simulink model "yunkongkaihuan"  (R2018a)
settings: Solver=VariableStepAuto  StartTime=0.0  StopTime=1  MaxStep=1e-5  RelTol=1e-3
values from neighbouring files (symbols this model uses):
  alpha = 0.05    [canshu.m]
  beta = 4.2    [canshu.m]
  IdN = 1.1    [canshu.m]
  Ki = (KI*taui*R)/(Ks*beta)    (= 0.193926092568)    [canshu.m]
  Kn = (h+1)*beta*Ce*Tm/(2*h*alpha*R*Tsigman)    (= 5.6)    [canshu.m]
  taui = Tl    (= 0.042)    [canshu.m]
  taun = h*Tsigman    (= 0.087)    [canshu.m]
  Toi = 0.002    [canshu.m]
  Ton = 0.01    [canshu.m]
  Ts = 0.00036    [canshu.m]
  UN = 220    [canshu.m]
libraries: powerlib x5, simulink x2
settings Model: Creator=pig head cookie  LastModifiedBy=lejmj

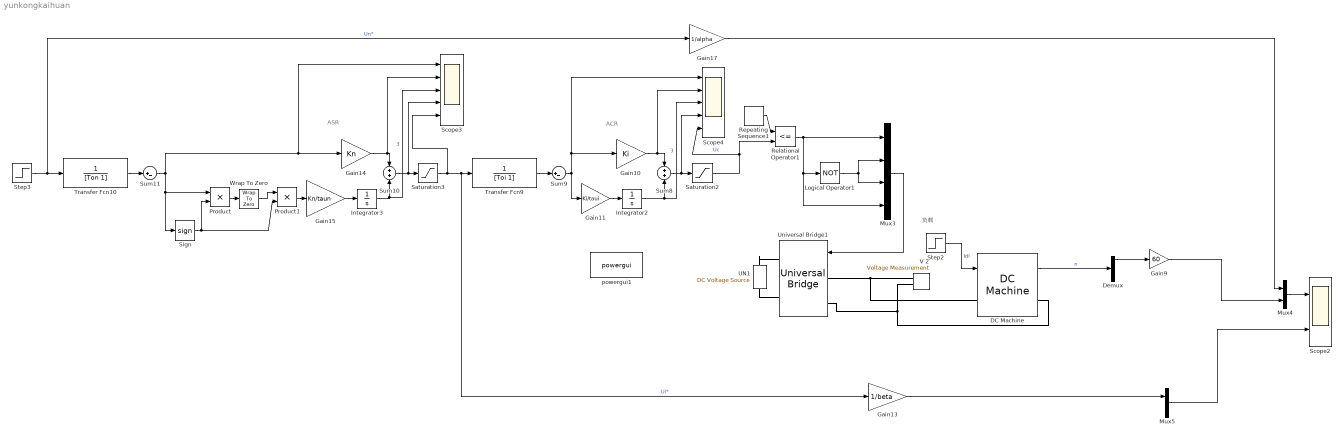
== system yunkongkaihuan ==
  note: ACR
  note: 负载
  note: ASR
  DC Machine : powerlib/Machines/DC Machine  PresetModel=No  MechanicalLoad=Torque TL  FieldType=Permanent magnet  ShowDetailedParameters=on  MeasurementBus=off  RLa="[2.06  0.0309]"  RLf="[ 240  120]"  Laf=1.8  MachineConstant=Back-emf constant (V/rpm)  Ke=0.12  Kt=1.8  J=0.1  Bm=0  Tf=0  w0=0.01  Ifinit=1  TsPowergui=0  TsBlock=-1
  Demux : Demux
  Gain10 : Gain  Gain=Ki
  Gain11 : Gain  Gain=Ki/taui
  Gain13 : Gain  Gain=1/beta
  Gain14 : Gain  Gain=Kn
  Gain15 : Gain  Gain=Kn/taun
  Gain17 : Gain  Gain=1/alpha
  Gain9 : Gain  Gain=60
  Integrator2 : Integrator  LimitOutput=on  UpperSaturationLimit=12  LowerSaturationLimit=-12
  Integrator3 : Integrator  LimitOutput=on  UpperSaturationLimit=12  LowerSaturationLimit=-12
  Logical Operator1 : Logic  Operator=NOT  AllPortsSameDT=off  OutDataTypeStr=boolean
  Mux3 : Mux
  Mux4 : Mux  Inputs=2
  Mux5 : Mux  Inputs=2
  Product : Product
  Product1 : Product
  Relational Operator1 : RelationalOperator  Operator=<=  OutDataTypeStr=boolean  RndMeth=Simplest
  Repeating Sequence1 : simulink/Sources/Repeating Sequence  rep_seq_t=[0 Ts]  rep_seq_y=[-10 10]
  Saturation2 : Saturate  UpperLimit=10  LowerLimit=-10
  Saturation3 : Saturate  UpperLimit=10  LowerLimit=-10
  Scope2 : Scope  NumInputPorts=2
  Scope3 : Scope  NumInputPorts=5
  Scope4 : Scope  NumInputPorts=5
  Sign : Signum
  Step2 : Step  Time=0.1  After=IdN  SampleTime=0
  Step3 : Step  Time=0.1  SampleTime=0
  Sum10 : Sum  Inputs=+|+
  Sum11 : Sum  Inputs=|+-
  Sum8 : Sum  Inputs=+|+
  Sum9 : Sum  Inputs=|+-
  Transfer Fcn10 : TransferFcn  Denominator=[Ton 1]
  Transfer Fcn9 : TransferFcn  Denominator=[Toi 1]
  UN1 : powerlib/Electrical Sources/DC Voltage Source  Amplitude=UN  Measurements=None
  Universal Bridge1 : powerlib/Power Electronics/Universal Bridge  Arms=2  SnubberResistance=1e5  SnubberCapacitance=inf  Device=IGBT / Diodes  Ron=1e-3  Lon=0  ForwardVoltages="[  0  0  ]"  ForwardVoltage=0  GTOparameters=[ 10e-6 , 20e-6 ]  IGBTparameters=[ 1e-6 , 2e-6 ]  Measurements=None  Measurements_2=None  converterType=Rectifier
  V 2 : powerlib/Measurements/Voltage Measurement  PhasorSimulation=off  OutputType=Complex  PSBequivalent=0
  Wrap To Zero : simulink/Discontinuities/Wrap To Zero  Threshold=5
      settings: SourceProductName=Simulink  SourceProductBaseCode=SL
  powergui1 : powerlib/powergui  Priority=1  SimulationMode=Continuous  SampleTime=50e-6  frequency=60  Iterations=50  frequencyindice=0  Pbase=100e6  ErrMax=1e-4  UnitsV=kV  UnitsW=MW  buscounter=0  FunctionMessages=off  echomessages=off  EnableUseOfTLC=off  CurrentSourceSwitches=off  DisableSnubberDevices=off  DisableRonSwitches=off  DisableVfSwitches=off  DisplayEquations=off  SolverType=Tustin/Backward Euler (TBE)  Interpol=off  ExternalGateDelay=off  methode=off  Ts=100  x0status=blocks  SPID=on  SwTol=0  HookPort=off  RestoreLinks=warning  ResistiveCurrentMeasurement=off  Frange=[0:2:500]  Ylog=off  Xlog=on  ShowGrid=off  save=off  variable=ZData  structure=0  ZoomFFT=off  StartTime=0.0  cycles=1  DisplayStyle=1  fundamental=60  FreqAxis=off  MaxFrequency=1000  frequencyindicesteady=1  RmsSteady=1  display=off
  wires:
  Step3/1 -> Gain17/1, Transfer Fcn10/1  "Un*"
  Mux3/1 -> Universal Bridge1/1
  Integrator2/1 -> Scope4/3, Sum8/2  "3"
  Transfer Fcn9/1 -> Sum9/1
  Saturation2/1 -> Scope4/5, Relational Operator1/2  "Uc"
  Sum8/1 -> Scope4/4, Saturation2/1
  Mux5/1 -> Scope2/2
  Mux4/1 -> Scope2/1
  Saturation3/1 -> Scope3/5, Gain13/1, Transfer Fcn9/1  "Ui*"
  Sum10/1 -> Scope3/4, Saturation3/1
  Gain15/1 -> Integrator3/1
  Integrator3/1 -> Scope3/3, Sum10/2  "3"
  Sum11/1 -> Scope3/1, Gain14/1, Product/1, Sign/1
  Gain11/1 -> Integrator2/1
  Relational Operator1/1 -> Mux3/4, Logical Operator1/1, Mux3/1
  Transfer Fcn10/1 -> Sum11/1
  Repeating Sequence1/1 -> Relational Operator1/1
  Gain10/1 -> Scope4/2, Sum8/1
  Gain14/1 -> Scope3/2, Sum10/1
  Sum9/1 -> Gain10/1, Scope4/1, Gain11/1
  Gain13/1 -> Mux5/1
  Gain17/1 -> Mux4/1
  Logical Operator1/1 -> Mux3/2, Mux3/3
  DC Machine/1 -> Demux/1  "n"
  Demux/1 -> Gain9/1
  Gain9/1 -> Mux4/2
  Step2/1 -> DC Machine/1  "Idl"
  Sign/1 -> Product1/2, Product/2
  Product/1 -> Wrap To Zero/1
  Wrap To Zero/1 -> Product1/1
  Product1/1 -> Gain15/1
  connections:
  UN1/RConn1 -- Universal Bridge1/RConn1
  Universal Bridge1/LConn1 -- V 2/LConn1 -- DC Machine/LConn1
  UN1/LConn1 -- Universal Bridge1/RConn2
  V 2/LConn2 -- Universal Bridge1/LConn2 -- DC Machine/RConn1
